simulink model "RobotArm_PickAndPlace"  (R2021a)
settings: Solver=VariableStepAuto  StartTime=0.0  StopTime=10.0  RelTol=1e-3
InitFcn:
  | cameraPoints=[0.1 0.1; 0.2 -0.2; 0.05 0.05];
  | InitPoint=[0.2452; 0; 0.2562];
libraries: arduinolib x13
settings Model: Creator=loris  LastModifiedBy=loris

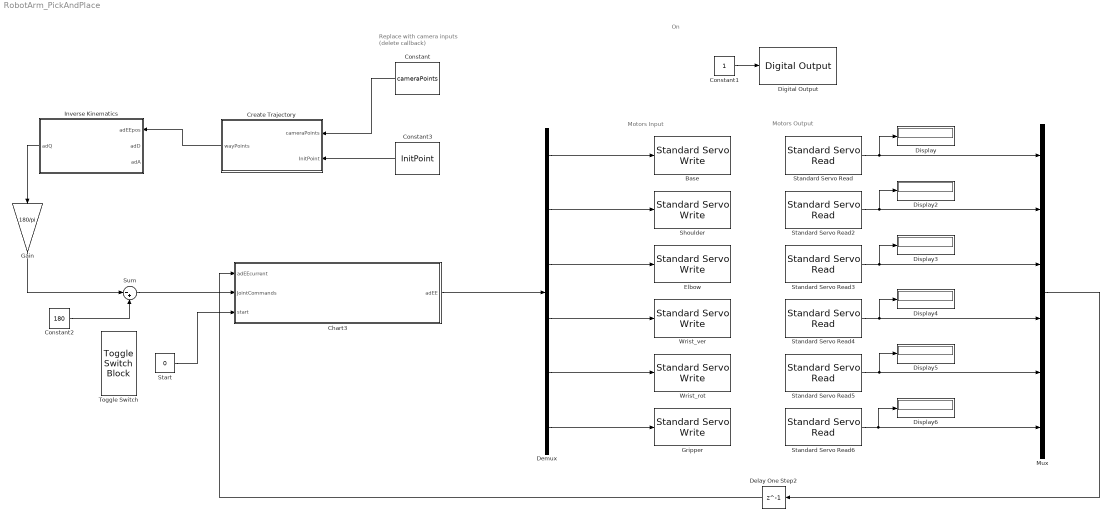
== system RobotArm_PickAndPlace ==
  note: Replace with camera inputs
      | (delete callback)
  note: On
  note: Motors Output
  note: Motors Input
  Base : arduinolib/Standard Servo Write  pinNumber=11  ServoIndex=0  blockPlatform=ARDUINO
  Chart3 : Stateflow chart  TreatAsAtomicUnit=on  SystemSampleTime=0.02
  Constant : Constant  Value=cameraPoints
  Constant1 : Constant
  Constant2 : Constant  Value=180
  Constant3 : Constant  Value=InitPoint
  Create Trajectory : MATLAB Function  TreatAsAtomicUnit=on
  Delay One Step2 : Delay  DelayLength=1  InitialCondition=[90; 90; 90; 90; 0; 0]
  Demux : Demux  Outputs=6
  Digital Output : arduinolib/Digital Output  pinNumber=12  Direction=output  blockPlatform=arduino
  Display{,2..6} (6 alike) : Display
  Elbow : arduinolib/Standard Servo Write  pinNumber=9  ServoIndex=1  blockPlatform=ARDUINO
  Gain : Gain  Gain=180/pi
  Gripper : arduinolib/Standard Servo Write  pinNumber=3  ServoIndex=2  blockPlatform=ARDUINO
  Inverse Kinematics : MATLAB Function  TreatAsAtomicUnit=on
  Mux : Mux  Inputs=6
  Shoulder : arduinolib/Standard Servo Write  pinNumber=10  ServoIndex=3  blockPlatform=ARDUINO
  Standard Servo Read : arduinolib/Standard Servo Read  pinNumber=11  SampleTime=0.02  ServoIndex=0  blockPlatform=ARDUINO
      settings: SourceProductBaseCode=ARDUINO
  Standard Servo Read2 : arduinolib/Standard Servo Read  pinNumber=10  SampleTime=0.02  ServoIndex=3  blockPlatform=ARDUINO
      settings: SourceProductBaseCode=ARDUINO
  Standard Servo Read3 : arduinolib/Standard Servo Read  pinNumber=9  SampleTime=0.02  ServoIndex=1  blockPlatform=ARDUINO
      settings: SourceProductBaseCode=ARDUINO
  Standard Servo Read4 : arduinolib/Standard Servo Read  pinNumber=6  SampleTime=0.02  ServoIndex=4  blockPlatform=ARDUINO
      settings: SourceProductBaseCode=ARDUINO
  Standard Servo Read5 : arduinolib/Standard Servo Read  pinNumber=5  SampleTime=0.02  ServoIndex=5  blockPlatform=ARDUINO
      settings: SourceProductBaseCode=ARDUINO
  Standard Servo Read6 : arduinolib/Standard Servo Read  pinNumber=3  SampleTime=0.02  ServoIndex=2  blockPlatform=ARDUINO
      settings: SourceProductBaseCode=ARDUINO
  Start : Constant  Value=0
  Sum : Sum  Inputs=|-+
  Toggle Switch : ToggleSwitchBlock  LabelPosition=Hide
      settings: Values={{'Off', 'On'}, [0 1]}
  Wrist_rot : arduinolib/Standard Servo Write  pinNumber=5  ServoIndex=5  blockPlatform=ARDUINO
  Wrist_ver : arduinolib/Standard Servo Write  pinNumber=6  ServoIndex=4  blockPlatform=ARDUINO
  wires:
  Constant1/1 -> Digital Output/1
  Demux/4 -> Wrist_ver/1
  Demux/1 -> Base/1
  Chart3/1(adEE) -> Demux/1
  Demux/3 -> Elbow/1
  Demux/2 -> Shoulder/1
  Standard Servo Read5/1 -> Display5/1, Mux/5
  Standard Servo Read6/1 -> Display6/1, Mux/6
  Standard Servo Read4/1 -> Display4/1, Mux/4
  Standard Servo Read/1 -> Display/1, Mux/1
  Standard Servo Read2/1 -> Display2/1, Mux/2
  Delay One Step2/1 -> Chart3/1(adEEcurrent)
  Demux/6 -> Gripper/1
  Mux/1 -> Delay One Step2/1
  Standard Servo Read3/1 -> Display3/1, Mux/3
  Demux/5 -> Wrist_rot/1
  Constant/1 -> Create Trajectory/1(cameraPoints)
  Create Trajectory/1(wayPoints) -> Inverse Kinematics/1(adEEpos)
  Constant3/1 -> Create Trajectory/2(InitPoint)
  Start/1 -> Chart3/3(start)
  Sum/1 -> Chart3/2(JointCommands)
  Inverse Kinematics/1(adQ) -> Gain/1
  Constant2/1 -> Sum/2
  Gain/1 -> Sum/1

== stateflow chart RobotArm_PickAndPlace/Chart3 ==
  settings: executeAtInitialization=1
  state ToNextState
    entry:
    if currentState<size(JointCommands,1)
    currentState=currentState+1;
    else
    stop=1;
    end
    next=0;
    gripper=0;
  state WayPointReached
    entry:
    if currentState==1
    GripperDesired=50;
    elseif currentState==3
    GripperDesired=10;
    end
    during:
    adEE=[adEE(1:5);nextStep(adEEcurrent(6),GripperDesired)];
    gripper=CheckGripperReached(adEEcurrent(6),GripperDesired)
  state Init
    entry:
    currentState=1;
    next=0;
    stop=0;
    gripper=0;
    GripperDesired=10;
    adEE=[90; 90; 45; 45; 0; 10];
  state WaitingForCamera
    entry:
    stop=0;
  state ToNextPoint
    during:
    adEE = [
    nextStep(adEEcurrent(1), adEEdesired(1));
    nextStep(adEEcurrent(2), adEEdesired(2));
    nextStep(adEEcurrent(3), adEEdesired(3));
    nextStep(adEEcurrent(4), adEEdesired(4));
    nextStep(adEEcurrent(5), adEEdesired(5));
    nextStep(adEEcurrent(6), adEEdesired(6))];
    next=CheckWayPointReached(adEEcurrent, adEEdesired);
  state SetEEDesired
    entry:
    adEEdesired=JointCommands(currentState,:)';
  (default) -> Init
  WayPointReached -> ToNextState : [gripper==1]
  ToNextState -> WaitingForCamera [order 2] : [stop==1]
  ToNextState -> SetEEDesired [order 1] : [stop==0]
  Init -> WaitingForCamera
  ToNextPoint -> WayPointReached : [next==1]
  WaitingForCamera -> SetEEDesired : [start==1]
  SetEEDesired -> ToNextPoint
  data: current function_input; desired function_input; v function_output; current function_input; desired function_input; gripper function_output; current function_input; desired function_input; v function_output; current function_input; desired function_input; next function_output; adEEcurrent input; adEE output; adEEdesired local; currentState local; JointCommands input; next local; stop local; start input; GripperDesired local; gripper local
  function v = nextStep(current, desired):
    | function v = nextStep(current, desired)
    | if (current < desired)
    |     current = current + 1;
    | end
    | 
    | if (current > desired)
    |     current = current - 1;
    | end
    | 
    | v = current;
    | end
  function gripper = CheckGripperReached(current, desired):
    | function gripper = CheckGripperReached(current, desired)
    |     check=current-desired;
    |     if check==0
    |         gripper=1;
    |     else
    |         gripper=0;
    |     end
    | end
  function v = nextStep(current, desired):
    | function v = nextStep(current, desired)
    | if (current < desired)
    |     current = current + 1;
    | end
    | 
    | if (current > desired)
    |     current = current - 1;
    | end
    | 
    | v = current;
    | end
  function next = CheckWayPointReached(current, desired):
    | function next = CheckWayPointReached(current, desired)
    |     check=current-desired;
    |     if norm(check,2)<0.005
    |         next=1;
    |     else
    |         next=0;
    |     end
    | end

== matlab function RobotArm_PickAndPlace/Create Trajectory ==
  data: cameraPoints input; wayPoints output; InitPoint input
function wayPoints = fcn(cameraPoints, InitPoint)
    if size(cameraPoints,1)>0
        wayPoints=[cameraPoints(:,1), InitPoint, cameraPoints(:,2), InitPoint];
    else
        return
    end
end

== matlab function RobotArm_PickAndPlace/Inverse Kinematics ==
  data: adEEpos input; adQ output; adD input; adA input
function adQ = fIKIN(adEEpos, adD, adA)
%{
    @brief      Compute the Joint configuration from EE position.
    @details    Joint Configuration is computed with geometric
                considerations.
    
    @param      adEEpos: (x; y; z) desired EE position
    @param      adD:     distance between O_i-1 and O'           (5, 1)
    @param      adA:     distance signless between z_i-1 and z_i (5, 1)

    @return     adQ:     joints configuration (5, 1)   
%}

adQ = [pi/2; pi/2; pi/2; pi/2; 0];   % Home

% Check for dimensions
if(size(adEEpos, 1) == 1 && size(adEEpos, 2) == 3)
    adEEpos = adEEpos';
end

% Test to handle wrong input
if(size(adEEpos, 1) ~= 3 && size(adEEpos, 2) ~= 1)
    return;
end

% Verify (point in Robot WS)
if (fIsInsideWorkspace(adEEpos, 435, 80, 220) == false)
    return;
end

%%% Azimuth and Elevation
dAzRad  = atan2(adEEpos(2), adEEpos(1));
dPhiRad = atan2(adEEpos(3), sqrt(adEEpos(1)^2 + adEEpos(2)^2));

%%% Desired Coordinates
dWx     = sqrt(adEEpos(1)^2 + adEEpos(2)^2) - (adA(4) * cos(dPhiRad));
dWz     = (adEEpos(3) - adD(1)) - (adA(4) * sin(dPhiRad));

%%% Computation
% Base
q1  = dAzRad;

% Elbow
c3      = (dWx^2 + dWz^2 - adA(2)^2 - adA(3)^2) / (2 * adA(2) * adA(3));
s3      = -sqrt(1 - c3^2);
q3      = atan2(s3, c3);

% Shoulder
% c2 = (dWx * (adA(2) + adA(3) * c3) + dWz * adA(3) * s3) / (dWx^2 + dWz^2);
% s2 = (dWz * (adA(2) + adA(3) * c3) + dWx * adA(3) * s3) / (dWx^2 + dWz^2);
% q2 = atan2(s2, c2);
beta    = atan2(adA(3) * s3, adA(2) + adA(3) * c3);
gamma   = atan2(dWz, dWx);
q2      = gamma - beta;

% Wrist
q4 = dPhiRad - q2 - q3;

% Mapping Motors
%adQ = [pi/2 - q1; q2; q3 + pi/2; q4 + pi/2; 0];
adQ     = [q1; q2; q3; q4; 0];

end
